simulink model "ES259A_BattVltgCorrln"  (R2013b)
settings: Solver=FixedStepDiscrete  SolverMode=SingleTasking  StartTime=0.0  StopTime=Inf  FixedStep=0.002  RelTol=1e-3
values from neighbouring files (symbols this model uses):
  BattVltgCorrlnAllwdVltgDif = DataDict.Calibration    [ES259A_BattVltgCorrln_DataDict.m]
  BattVltgCorrlnBattLoVltg = DataDict.Calibration    [ES259A_BattVltgCorrln_DataDict.m]
  BattVltgCorrlnBattOverVltg = DataDict.Calibration    [ES259A_BattVltgCorrln_DataDict.m]
  BattVltgCorrlnBattUnderVltg = DataDict.Calibration    [ES259A_BattVltgCorrln_DataDict.m]
  BattVltgCorrlnNtc0x03C0x0440x04CFailStep = DataDict.Calibration    [ES259A_BattVltgCorrln_DataDict.m]
  BattVltgCorrlnNtc0x03C0x0440x04CPassStep = DataDict.Calibration    [ES259A_BattVltgCorrln_DataDict.m]
  BattVltgCorrlnNtc0x03DFailStep = DataDict.Calibration    [ES259A_BattVltgCorrln_DataDict.m]
  BattVltgCorrlnNtc0x03DPassStep = DataDict.Calibration    [ES259A_BattVltgCorrln_DataDict.m]
  BattVltgCorrlnNtc0x0B0FailStep = DataDict.Calibration    [ES259A_BattVltgCorrln_DataDict.m]
  BattVltgCorrlnNtc0x0B0PassStep = DataDict.Calibration    [ES259A_BattVltgCorrln_DataDict.m]
  BattVltgCorrlnNtc0x0B1FailStep = DataDict.Calibration    [ES259A_BattVltgCorrln_DataDict.m]
  BattVltgCorrlnNtc0x0B1PassStep = DataDict.Calibration    [ES259A_BattVltgCorrln_DataDict.m]
  BattVltgCorrlnNtc0x0B5FailStep = DataDict.Calibration    [ES259A_BattVltgCorrln_DataDict.m]
  BattVltgCorrlnNtc0x0B5PassStep = DataDict.Calibration    [ES259A_BattVltgCorrln_DataDict.m]
  BattVltgCorrlnRcvrlBattLoVltg = DataDict.Calibration    [ES259A_BattVltgCorrln_DataDict.m]
  BattVltgCorrlnRcvrlBattOverVltg = DataDict.Calibration    [ES259A_BattVltgCorrln_DataDict.m]
  BattVltgCorrlnRcvrlBattUnderVltg = DataDict.Calibration    [ES259A_BattVltgCorrln_DataDict.m]
  BattVltgCorrlnSysMinVltg = DataDict.ImprtdCal    [ES250A_BattVltg_DataDict.m]    (also in ES259A_BattVltgCorrln_DataDict.m = DataDict.Calibration)
  BattVltgSwdMax = DataDict.Calibration    [ES250A_BattVltg_DataDict.m]
  ELECGLBPRM_STRTUPSTPWRDISCNCTBTESTCMPL_CNT_U08 = DataDict.Constant    [ES999A_ElecGlbPrm_DataDict.m]
  SYSVLTGFLTDUALIVTR_CNT_U08 = DataDict.Constant    [ES259A_BattVltgCorrln_DataDict.m]
undefined symbols (not defined in the file or in its folder): NtcNr1, NtcSts1, SigQlfr1
libraries: simulink x14
(part 7 of 7)

== stateflow chart ES259A_BattVltgCorrln/BattVltgCorrln/BattVltgCorrlnPer1/Battery Voltage Diagnostics/Inhibition Off/UnderVltg <= BattVltg < LowVltg/If Action 1/SetNtcStsB5/ISO Fault Debounce Design NOT TO BE IMPLEMENTED IN THIS FDD USED ONLY FOR SIMULATION PURPOSES ==
  note: NTCSTS_PASSD           (0)
      | NTCSTS_FAILD             (1)
      | NTCSTS_PREPASSD   (2)
      | NTCSTS_PREFAILD     (3)
      |
      | SIGQLFR_NORES        (0)
      | SIGQLFR_PASSD         (1)
      | SIGQLFR_FAILD           (2)
  note: Fail step Loop
  note: Pass step Loop
  note: 
  (default) -> (junction 89)
  (junction 89) -> (junction 95) [order 1] : [NtcSts == 3]
  (junction 89) -> (junction 93) [order 2] : [ NtcSts == 2]
  (junction 93) -> (junction 230) [order 2] : {
      | DebCntr = DebCntr - DebStep;
      | }
  (junction 95) -> (junction 216) [order 2] : [DebCntr <= 0]
      | {
      | DebCntr = DebStep;
      | }
  (junction 95) -> (junction 103) [order 1] : [DebCntr > 0]
  (junction 93) -> (junction 123) [order 1] : [(DebCntr - DebStep) <= -32768]
      | {
      | DebCntr = -32768;
      | Qualifier = 1;
      | }
  (junction 230) -> (junction 231)
  (junction 103) -> (junction 216) [order 2] : {
      | DebCntr = DebCntr + DebStep;
      | }
  (junction 216) -> (junction 220) [order 2]
  (junction 216) -> (junction 220) [order 1] : [(DebCntr + DebStep) >=32767]
      | {
      | DebCntr = 32767;
      | Qualifier =2;
      | }
  (junction 103) -> (junction 220) [order 1] : [(DebCntr + DebStep) >=32767]
      | {
      | DebCntr = 32767;
      | Qualifier =2;
      | }
  (junction 220) -> (junction 141)
  (junction 123) -> (junction 141)
  (junction 231) -> (junction 123)
  (junction 141) -> (junction 159)
  data: NtcSts input uint8; Qualifier output uint8 =0; DebStep input uint16; DebCntr local int16

== stateflow chart ES259A_BattVltgCorrln/BattVltgCorrln/BattVltgCorrlnPer1/Battery Voltage Diagnostics/Inhibition Off/BattVltg < UnderVltg/SetNtcStsB0/ISO Fault Debounce Design NOT TO BE IMPLEMENTED IN THIS FDD USED ONLY FOR SIMULATION PURPOSES ==
  note: NTCSTS_PASSD           (0)
      | NTCSTS_FAILD             (1)
      | NTCSTS_PREPASSD   (2)
      | NTCSTS_PREFAILD     (3)
      |
      | SIGQLFR_NORES        (0)
      | SIGQLFR_PASSD         (1)
      | SIGQLFR_FAILD           (2)
  note: Fail step Loop
  note: Pass step Loop
  note: 
  (default) -> (junction 89)
  (junction 89) -> (junction 95) [order 1] : [NtcSts == 3]
  (junction 89) -> (junction 93) [order 2] : [ NtcSts == 2]
  (junction 93) -> (junction 230) [order 2] : {
      | DebCntr = DebCntr - DebStep;
      | }
  (junction 95) -> (junction 216) [order 2] : [DebCntr <= 0]
      | {
      | DebCntr = DebStep;
      | }
  (junction 95) -> (junction 103) [order 1] : [DebCntr > 0]
  (junction 93) -> (junction 123) [order 1] : [(DebCntr - DebStep) <= -32768]
      | {
      | DebCntr = -32768;
      | Qualifier = 1;
      | }
  (junction 230) -> (junction 231)
  (junction 103) -> (junction 216) [order 2] : {
      | DebCntr = DebCntr + DebStep;
      | }
  (junction 216) -> (junction 220) [order 2]
  (junction 216) -> (junction 220) [order 1] : [(DebCntr + DebStep) >=32767]
      | {
      | DebCntr = 32767;
      | Qualifier =2;
      | }
  (junction 103) -> (junction 220) [order 1] : [(DebCntr + DebStep) >=32767]
      | {
      | DebCntr = 32767;
      | Qualifier =2;
      | }
  (junction 220) -> (junction 141)
  (junction 123) -> (junction 141)
  (junction 231) -> (junction 123)
  (junction 141) -> (junction 159)
  data: NtcSts input uint8; Qualifier output uint8 =0; DebStep input uint16; DebCntr local int16

== stateflow chart ES259A_BattVltgCorrln/BattVltgCorrln/BattVltgCorrlnPer1/Battery Voltage Diagnostics/Inhibition Off/BattVltg < UnderVltg/SetNtcStsB1/ISO Fault Debounce Design NOT TO BE IMPLEMENTED IN THIS FDD USED ONLY FOR SIMULATION PURPOSES ==
  note: NTCSTS_PASSD           (0)
      | NTCSTS_FAILD             (1)
      | NTCSTS_PREPASSD   (2)
      | NTCSTS_PREFAILD     (3)
      |
      | SIGQLFR_NORES        (0)
      | SIGQLFR_PASSD         (1)
      | SIGQLFR_FAILD           (2)
  note: Fail step Loop
  note: Pass step Loop
  note: 
  (default) -> (junction 89)
  (junction 89) -> (junction 95) [order 1] : [NtcSts == 3]
  (junction 89) -> (junction 93) [order 2] : [ NtcSts == 2]
  (junction 93) -> (junction 230) [order 2] : {
      | DebCntr = DebCntr - DebStep;
      | }
  (junction 95) -> (junction 216) [order 2] : [DebCntr <= 0]
      | {
      | DebCntr = DebStep;
      | }
  (junction 95) -> (junction 103) [order 1] : [DebCntr > 0]
  (junction 93) -> (junction 123) [order 1] : [(DebCntr - DebStep) <= -32768]
      | {
      | DebCntr = -32768;
      | Qualifier = 1;
      | }
  (junction 230) -> (junction 231)
  (junction 103) -> (junction 216) [order 2] : {
      | DebCntr = DebCntr + DebStep;
      | }
  (junction 216) -> (junction 220) [order 2]
  (junction 216) -> (junction 220) [order 1] : [(DebCntr + DebStep) >=32767]
      | {
      | DebCntr = 32767;
      | Qualifier =2;
      | }
  (junction 103) -> (junction 220) [order 1] : [(DebCntr + DebStep) >=32767]
      | {
      | DebCntr = 32767;
      | Qualifier =2;
      | }
  (junction 220) -> (junction 141)
  (junction 123) -> (junction 141)
  (junction 231) -> (junction 123)
  (junction 141) -> (junction 159)
  data: NtcSts input uint8; Qualifier output uint8 =0; DebStep input uint16; DebCntr local int16

== stateflow chart ES259A_BattVltgCorrln/BattVltgCorrln/BattVltgCorrlnPer1/Battery Voltage Diagnostics/Inhibition Off/BattVltg < UnderVltg/SetNtcStsB5/ISO Fault Debounce Design NOT TO BE IMPLEMENTED IN THIS FDD USED ONLY FOR SIMULATION PURPOSES ==
  note: NTCSTS_PASSD           (0)
      | NTCSTS_FAILD             (1)
      | NTCSTS_PREPASSD   (2)
      | NTCSTS_PREFAILD     (3)
      |
      | SIGQLFR_NORES        (0)
      | SIGQLFR_PASSD         (1)
      | SIGQLFR_FAILD           (2)
  note: Fail step Loop
  note: Pass step Loop
  note: 
  (default) -> (junction 89)
  (junction 89) -> (junction 95) [order 1] : [NtcSts == 3]
  (junction 89) -> (junction 93) [order 2] : [ NtcSts == 2]
  (junction 93) -> (junction 230) [order 2] : {
      | DebCntr = DebCntr - DebStep;
      | }
  (junction 95) -> (junction 216) [order 2] : [DebCntr <= 0]
      | {
      | DebCntr = DebStep;
      | }
  (junction 95) -> (junction 103) [order 1] : [DebCntr > 0]
  (junction 93) -> (junction 123) [order 1] : [(DebCntr - DebStep) <= -32768]
      | {
      | DebCntr = -32768;
      | Qualifier = 1;
      | }
  (junction 230) -> (junction 231)
  (junction 103) -> (junction 216) [order 2] : {
      | DebCntr = DebCntr + DebStep;
      | }
  (junction 216) -> (junction 220) [order 2]
  (junction 216) -> (junction 220) [order 1] : [(DebCntr + DebStep) >=32767]
      | {
      | DebCntr = 32767;
      | Qualifier =2;
      | }
  (junction 103) -> (junction 220) [order 1] : [(DebCntr + DebStep) >=32767]
      | {
      | DebCntr = 32767;
      | Qualifier =2;
      | }
  (junction 220) -> (junction 141)
  (junction 123) -> (junction 141)
  (junction 231) -> (junction 123)
  (junction 141) -> (junction 159)
  data: NtcSts input uint8; Qualifier output uint8 =0; DebStep input uint16; DebCntr local int16

== stateflow chart ES259A_BattVltgCorrln/BattVltgCorrln/BattVltgCorrlnPer1/Battery Voltage Diagnostics/Inhibition Off/LowVltg <= Batt <= OverVltg/If Action/SetNtcStsB0/ISO Fault Debounce Design NOT TO BE IMPLEMENTED IN THIS FDD USED ONLY FOR SIMULATION PURPOSES ==
  note: NTCSTS_PASSD           (0)
      | NTCSTS_FAILD             (1)
      | NTCSTS_PREPASSD   (2)
      | NTCSTS_PREFAILD     (3)
      |
      | SIGQLFR_NORES        (0)
      | SIGQLFR_PASSD         (1)
      | SIGQLFR_FAILD           (2)
  note: Fail step Loop
  note: Pass step Loop
  note: 
  (default) -> (junction 89)
  (junction 89) -> (junction 95) [order 1] : [NtcSts == 3]
  (junction 89) -> (junction 93) [order 2] : [ NtcSts == 2]
  (junction 93) -> (junction 230) [order 2] : {
      | DebCntr = DebCntr - DebStep;
      | }
  (junction 95) -> (junction 216) [order 2] : [DebCntr <= 0]
      | {
      | DebCntr = DebStep;
      | }
  (junction 95) -> (junction 103) [order 1] : [DebCntr > 0]
  (junction 93) -> (junction 123) [order 1] : [(DebCntr - DebStep) <= -32768]
      | {
      | DebCntr = -32768;
      | Qualifier = 1;
      | }
  (junction 230) -> (junction 231)
  (junction 103) -> (junction 216) [order 2] : {
      | DebCntr = DebCntr + DebStep;
      | }
  (junction 216) -> (junction 220) [order 2]
  (junction 216) -> (junction 220) [order 1] : [(DebCntr + DebStep) >=32767]
      | {
      | DebCntr = 32767;
      | Qualifier =2;
      | }
  (junction 103) -> (junction 220) [order 1] : [(DebCntr + DebStep) >=32767]
      | {
      | DebCntr = 32767;
      | Qualifier =2;
      | }
  (junction 220) -> (junction 141)
  (junction 123) -> (junction 141)
  (junction 231) -> (junction 123)
  (junction 141) -> (junction 159)
  data: NtcSts input uint8; Qualifier output uint8 =0; DebStep input uint16; DebCntr local int16

== stateflow chart ES259A_BattVltgCorrln/BattVltgCorrln/BattVltgCorrlnPer1/Battery Voltage Diagnostics/Inhibition Off/LowVltg <= Batt <= OverVltg/If Action 1/SetNtcStsB0/ISO Fault Debounce Design NOT TO BE IMPLEMENTED IN THIS FDD USED ONLY FOR SIMULATION PURPOSES ==
  note: NTCSTS_PASSD           (0)
      | NTCSTS_FAILD             (1)
      | NTCSTS_PREPASSD   (2)
      | NTCSTS_PREFAILD     (3)
      |
      | SIGQLFR_NORES        (0)
      | SIGQLFR_PASSD         (1)
      | SIGQLFR_FAILD           (2)
  note: Fail step Loop
  note: Pass step Loop
  note: 
  (default) -> (junction 89)
  (junction 89) -> (junction 95) [order 1] : [NtcSts == 3]
  (junction 89) -> (junction 93) [order 2] : [ NtcSts == 2]
  (junction 93) -> (junction 230) [order 2] : {
      | DebCntr = DebCntr - DebStep;
      | }
  (junction 95) -> (junction 216) [order 2] : [DebCntr <= 0]
      | {
      | DebCntr = DebStep;
      | }
  (junction 95) -> (junction 103) [order 1] : [DebCntr > 0]
  (junction 93) -> (junction 123) [order 1] : [(DebCntr - DebStep) <= -32768]
      | {
      | DebCntr = -32768;
      | Qualifier = 1;
      | }
  (junction 230) -> (junction 231)
  (junction 103) -> (junction 216) [order 2] : {
      | DebCntr = DebCntr + DebStep;
      | }
  (junction 216) -> (junction 220) [order 2]
  (junction 216) -> (junction 220) [order 1] : [(DebCntr + DebStep) >=32767]
      | {
      | DebCntr = 32767;
      | Qualifier =2;
      | }
  (junction 103) -> (junction 220) [order 1] : [(DebCntr + DebStep) >=32767]
      | {
      | DebCntr = 32767;
      | Qualifier =2;
      | }
  (junction 220) -> (junction 141)
  (junction 123) -> (junction 141)
  (junction 231) -> (junction 123)
  (junction 141) -> (junction 159)
  data: NtcSts input uint8; Qualifier output uint8 =0; DebStep input uint16; DebCntr local int16

== stateflow chart ES259A_BattVltgCorrln/BattVltgCorrln/BattVltgCorrlnPer1/Battery Voltage Diagnostics/Inhibition Off/LowVltg <= Batt <= OverVltg/No Fault Condition/SetNtcStsB0/ISO Fault Debounce Design NOT TO BE IMPLEMENTED IN THIS FDD USED ONLY FOR SIMULATION PURPOSES ==
  note: NTCSTS_PASSD           (0)
      | NTCSTS_FAILD             (1)
      | NTCSTS_PREPASSD   (2)
      | NTCSTS_PREFAILD     (3)
      |
      | SIGQLFR_NORES        (0)
      | SIGQLFR_PASSD         (1)
      | SIGQLFR_FAILD           (2)
  note: Fail step Loop
  note: Pass step Loop
  note: 
  (default) -> (junction 89)
  (junction 89) -> (junction 95) [order 1] : [NtcSts == 3]
  (junction 89) -> (junction 93) [order 2] : [ NtcSts == 2]
  (junction 93) -> (junction 230) [order 2] : {
      | DebCntr = DebCntr - DebStep;
      | }
  (junction 95) -> (junction 216) [order 2] : [DebCntr <= 0]
      | {
      | DebCntr = DebStep;
      | }
  (junction 95) -> (junction 103) [order 1] : [DebCntr > 0]
  (junction 93) -> (junction 123) [order 1] : [(DebCntr - DebStep) <= -32768]
      | {
      | DebCntr = -32768;
      | Qualifier = 1;
      | }
  (junction 230) -> (junction 231)
  (junction 103) -> (junction 216) [order 2] : {
      | DebCntr = DebCntr + DebStep;
      | }
  (junction 216) -> (junction 220) [order 2]
  (junction 216) -> (junction 220) [order 1] : [(DebCntr + DebStep) >=32767]
      | {
      | DebCntr = 32767;
      | Qualifier =2;
      | }
  (junction 103) -> (junction 220) [order 1] : [(DebCntr + DebStep) >=32767]
      | {
      | DebCntr = 32767;
      | Qualifier =2;
      | }
  (junction 220) -> (junction 141)
  (junction 123) -> (junction 141)
  (junction 231) -> (junction 123)
  (junction 141) -> (junction 159)
  data: NtcSts input uint8; Qualifier output uint8 =0; DebStep input uint16; DebCntr local int16
